simulink model "control_system"  (R2020b)
settings: Solver=FixedStepAuto  StartTime=0.0  StopTime=t_sim  FixedStep=Ts  RelTol=1e-2
values from neighbouring files (symbols this model uses):
  Hp = 10    [main_script.m]
  InitPosX = -2.4980e+03    (= -2498)    [main_script.m]
  InitPosY = -650.5503    [main_script.m]
  InitVelX = V0*cosd(InitYaw)    [main_script.m]
  InitVelY = V0*sind(InitYaw)    [main_script.m]
  InitYaw = 21    [main_script.m]
  lr = 1.592    [main_script.m]
  m = 1625    [main_script.m]
  Ts = 0.1    [main_script.m]
  V0 = 25    [main_script.m]
libraries: neural x856, simulink x1, autolibshared x1, drivingscenarioandsensors x1
(part 40 of 40)

== system control_system/HK con span dati 50 50 /Layer 3/Delays 1 ==
  "p{3}" : Inport  PortDimensions=50  SampleTime=0.1
      mask Display: e = 0.06;c1 = [120 230 180]/255;c2 = ([120 230 180]+0)/(256+128);c3 = ([120 230 180]+128)/(256+128);patch([0 1 1 0],[0 0 1 1],c1);patch([0 1 1 1-e 1-e 0+e],[0 0 1 1-e 0+e 0+e],c2);patch([0 0 1 1-e 0+e 0+e],[0 1 1 1-e 1-e 0+e],c3);plot([0 1 1 0 0],[0 0 1 1 0]);
  mux : Mux  Inputs=1
      mask Display: e = 0.06;c1 = [120 150 230]/255;c2 = ([120 150 230]+0)/383;c3 = ([120 150 230]+128)/383;patch([0 1 1 0],[0 0 1 1],c1);patch([0 1 1 1-e 1-e 0+e],[0 0 1 1-e 0+e 0+e],c2);patch([0 0 1 1-e 0+e 0+e],[0 1 1 1-e 1-e 0+e],c3);plot([0 1 1 0 0],[0 0 1 1 0]);disp('Mux')
  "pd{3,2}" : Outport
      mask Display: e = 0.06;c1 = [120 230 180]/255;c2 = ([120 230 180]+0)/(256+128);c3 = ([120 230 180]+128)/(256+128);patch([0 1 1 0],[0 0 1 1],c1);patch([0 1 1 1-e 1-e 0+e],[0 0 1 1-e 0+e 0+e],c2);patch([0 0 1 1-e 0+e 0+e],[0 1 1 1-e 1-e 0+e],c3);plot([0 1 1 0 0],[0 0 1 1 0]);
  wires:
  "p{3}"/1 -> mux/1
  mux/1 -> "pd{3,2}"/1

== system control_system/HK con span dati 50 50 /Layer 3/LW{3,2} ==
  "ad{3,2}" : Inport  PortDimensions=50  SampleTime=0.1
      mask Display: e = 0.06;c1 = [120 230 180]/255;c2 = ([120 230 180]+0)/(256+128);c3 = ([120 230 180]+128)/(256+128);patch([0 1 1 0],[0 0 1 1],c1);patch([0 1 1 1-e 1-e 0+e],[0 0 1 1-e 0+e 0+e],c2);patch([0 0 1 1-e 0+e 0+e],[0 1 1 1-e 1-e 0+e],c3);plot([0 1 1 0 0],[0 0 1 1 0]);
  "IW{3,2}(1,:)'" : Constant  Value=[-3.53332826646673137105381101719103753566741943359375;0.291507037926716783271530175625230185687541961669921875;-0.353172688693744574184307793984771706163883209228515625;-1.6395166117947235218110790810897015035152435302734375;0.50878764421372524306974582941620610654354095458984375;-0.5480368977260765550596488537848927080631256103515625;0.552184856715687288897242979146540164947509765625;0.76081482289424140486033820707234553992748260498046875;0.370219705857955216909971341010532341897487640380859375;1.6866898293792775831434482824988663196563720703125;0.46041883039566100510597834727377630770206451416015625;0.293600086588905295759133196042967028915882110595703125;0.438868226588818688416182567380019463598728179931640625;0.71701414029024979068793754777288995683193206787109375;0.60074691622149301029054413447738625109195709228515625;0.360264149329229510509975398235837928950786590576171875;0.34807246412229553289563455109600909054279327392578125;0.1417371042032999628457190510744112543761730194091796875;0.2504625689834882873441301853745244443416595458984375;-0.37020479133339201371910576199297793209552764892578125;-0.346173859388357929578461380515363998711109161376953125;0.3405441513736524594690990852541290223598480224609375;-0.34088615645206521431731516713625751435756683349609375;-0.179812084794879201155026748892851173877716064453125;0.1998575322053002534250509825142216868698596954345703125;-0.2200538783486616078999276169270160607993602752685546875;1.640532886970199388798619111184962093830108642578125;0.186500178645137515420771023855195380747318267822265625;0.5071129724580607511796870312537066638469696044921875;0.08063920908443254764730312444953597150743007659912109375;-0.306927876349457673388343437181902118027210235595703125;0.6080823360766220986306507256813347339630126953125;0.2892945314898811570714087793021462857723236083984375;-0.1795861371313421661621845260015106759965419769287109375;0.3366900876707565881673644980764947831630706787109375;-0.60768828590126344746380482320091687142848968505859375;-0.1801845560207073759784179856069386005401611328125;0.20445768532080810242490542805171571671962738037109375;-0.311847366447380258680510678459540940821170806884765625;0.2158239417458625852841436199014424346387386322021484375;2.1907776163678907010989860282279551029205322265625;0.2482784684639368910641366028357879258692264556884765625;0.64184501918167813361293383422889746725559234619140625;0.37579121007342031202114185362006537616252899169921875;-0.21851869728468098497131677504512481391429901123046875;-0.2276966088677858379707430458438466303050518035888671875;-3.356449993447315538475095308967866003513336181640625;3.484749592622747638159808047930710017681121826171875;-1.8624140445228880569317198023782111704349517822265625;2.150511605753588018075106447213329374790191650390625]
      mask Display: e = 0.06;c1 = [120 150 230]/255;c2 = ([120 150 230]+0)/383;c3 = ([120 150 230]+128)/383;patch([0 1 1 0],[0 0 1 1],c1);patch([0 1 1 1-e 1-e 0+e],[0 0 1 1-e 0+e 0+e],c2);patch([0 0 1 1-e 0+e 0+e],[0 1 1 1-e 1-e 0+e],c3);plot([0 1 1 0 0],[0 0 1 1 0]);disp('weights');
  Mux : Mux  Inputs=1
      mask Display: e = 0.06;c1 = [120 150 230]/255;c2 = ([120 150 230]+0)/383;c3 = ([120 150 230]+128)/383;patch([0 1 1 0],[0 0 1 1],c1);patch([0 1 1 1-e 1-e 0+e],[0 0 1 1-e 0+e 0+e],c2);patch([0 0 1 1-e 0+e 0+e],[0 1 1 1-e 1-e 0+e],c3);plot([0 1 1 0 0],[0 0 1 1 0]);disp('Mux');
  dotprod1 : neural/Weight Functions/dotprod
  "lz{3,2}" : Outport
      mask Display: e = 0.06;c1 = [120 230 180]/255;c2 = ([120 230 180]+0)/(256+128);c3 = ([120 230 180]+128)/(256+128);patch([0 1 1 0],[0 0 1 1],c1);patch([0 1 1 1-e 1-e 0+e],[0 0 1 1-e 0+e 0+e],c2);patch([0 0 1 1-e 0+e 0+e],[0 1 1 1-e 1-e 0+e],c3);plot([0 1 1 0 0],[0 0 1 1 0]);
  wires:
  "IW{3,2}(1,:)'"/1 -> dotprod1/1
  "ad{3,2}"/1 -> dotprod1/2
  dotprod1/1 -> Mux/1
  Mux/1 -> "lz{3,2}"/1

== matlab function control_system/scenario and environment/Pack Ego Actor ==
  data: pos input; a output Bus: BusActors1Actors size=1; vel input; yaw input; yawRate input
function a = packEgo(pos,vel,yaw,yawRate)
% Pack ego information into a single ego actor bus
%
% Imoprtant note:
% Output is a bus of type BusActorsActors. This is the same bus used by the
% Scenario Reader to output an individual actor. If you change the
% output bus name of Scenario Reader change the output bus name here
% as well by clicking on 'Edit Data' in the menu above.

a = struct(...
    'ActorID',1,...
    'Position', [pos(1) pos(2) 0], ...
    'Velocity', [vel(1) vel(2) 0], ...
    'Roll', 0, ...
    'Pitch', 0, ...
    'Yaw', yaw, ...
    'AngularVelocity', [0 0 yawRate]);

== matlab function control_system/MATLAB Function2 ==
  data: lanes input; latOff_1 output; latOff_2 output; latOff_3 output; latOff_4 output
function [latOff_1,latOff_2,latOff_3,latOff_4] = fcn(lanes)

latOff_1 = lanes.LaneBoundaries(1).LateralOffset;
latOff_2 = lanes.LaneBoundaries(2).LateralOffset;
latOff_3 = lanes.LaneBoundaries(3).LateralOffset;
latOff_4 = lanes.LaneBoundaries(4).LateralOffset;

== matlab function control_system/MATLAB Function6 ==
  data: steer_ang_deg input; acc_pedal_perc output; acc_m_s2 input; brake_pedal_perc output; steer_wheel_deg output
function [acc_pedal_perc,brake_pedal_perc,steer_wheel_deg] = actuators(steer_ang_deg,acc_m_s2)

steer_ratio = 15;
max_acc = 2;
max_dec = 3;

steer_wheel_deg = steer_ang_deg*steer_ratio;

acc_pedal_perc = 0;
brake_pedal_perc = 0;

if acc_m_s2 >= 0
    acc_pedal_perc = abs(acc_m_s2/max_acc)*100;
else
    brake_pedal_perc = abs(acc_m_s2/max_dec)*100;
end

== matlab function control_system/MATLAB Function4 ==
  data: lane_info input; k_hook input; x0 input; LAT_state input; LON_state input; LaneDet input; ObjDet input; X_opt input; InLK output size=22; InHK output size=26; InOT output size=22; InRE output size=22; OutLK output size=2; OutHK output size=2; OutOT output size=2; OutRE output size=2; vdes input
function [InLK,InHK,InOT,InRE,OutLK,OutHK,OutOT,OutRE] = IO_NN( lane_info, k_hook, x0, ...
    LAT_state, LON_state, LaneDet,ObjDet,X_opt,vdes)

%% INITIALIZATION
% if the Net is disabled both Out and In are set to 0

N_line = 4-lane_info(1)+1;
Curv = LaneDet.LaneBoundaries(N_line).Curvature(end);

num_coord = 4:6;
nR = 22;%8+num_coord*4+1;
 
OutLK = zeros(2,1);
OutHK = zeros(2,1);
OutOT = zeros(2,1);
OutRE = zeros(2,1);

InLK = zeros(nR,1);
InHK = zeros(nR+4,1);
InOT = zeros(nR,1);
InRE = zeros(nR,1);

%% TAKING MEASURES
if lane_info(3) == 1
    if(lane_info(1) == lane_info(2))
        LL = 4-lane_info(2);
        RL = 4-lane_info(1)+2;
    else 
        LL = 4-lane_info(2);
        RL = 4-lane_info(1)+1;
    end
    
elseif lane_info(3) == -1
        if(lane_info(1) == lane_info(2))
            LL = 4-lane_info(1)-1;
            RL = 4-lane_info(2)+1;
        else
            LL = 4-lane_info(1);
            RL = 4-lane_info(2)+1;
        end
else
    LL = 4-lane_info(2);
    RL = 4-lane_info(1)+1;
end


wall_measures = [LaneDet.LaneBoundaries(LL).Coordinates(num_coord,1)
                 LaneDet.LaneBoundaries(LL).Coordinates(num_coord,2)
                 LaneDet.LaneBoundaries(RL).Coordinates(num_coord,1)
                 LaneDet.LaneBoundaries(RL).Coordinates(num_coord,2)];
             
if k_hook ~= 0        
    Obs_measures = [ObjDet.Actors(k_hook).Position(1);
                    ObjDet.Actors(k_hook).Position(2);
                    ObjDet.Actors(k_hook).Velocity(1);
                    ObjDet.Actors(k_hook).Velocity(2)];
else
    Obs_measures = zeros(4,1);
end


if LON_state == 2
    if LAT_state == 2
        % LANE KEEPING NN
        InLK = [x0;
                vdes;
                wall_measures;
                Curv];
        OutLK = [X_opt(1,1);
                 X_opt(1,2)];
            
%     elseif LAT_state == 3
%         % OVERTAKE NN
%         InOT = [x0;
%                 t0;
%                 wall_measures;
%                   Curv];
%         OutOT = [X_opt(1,1);
%                 X_opt(1,2)];
%             
%     elseif LAT_state == 4
%         % RE-ENTRY NN
%         InRE = [x0;
%                 t0;
%                 wall_measures;
%                   Curv];
%         OutRE = [X_opt(1,1);
%                 X_opt(1,2)];
    end
    
elseif LON_state == 3
    % HOOKING NN
    InHK = [x0;
            vdes;
            wall_measures;
            Obs_measures;
                  Curv];
    OutHK = [X_opt(1,1);
             X_opt(1,2)];
end

== matlab function control_system/MATLAB Function5 ==
  data: LatState input; LonState input; en1 output; en2 output; en3 output; en4 output
function [en1,en2,en3,en4] = enable_funct(LatState,LonState)
% Finite-state machine for the lateral dynamics

% states:       "IDLE"  = [0]do nothing
%                "RST"  = [1]reset variables
%       "lane_keeping"  = [2]Lane keeping 
%         "overtaking"  = [3]move in the next left lane
%           "re_entry"  = [4]move in the next right lane

% Finite-state machine for the longitudinal dynamics

% states:       "IDLE"  = [0]do nothing
%                "RST"  = [1]reset variables
%           "vel_cntr"  = [2]velocity control
%            "hooking"  = [3]spacing control

en1 = 0;
en2 = 0;
en3 = 0;
en4 = 0;

if(LatState == 2 && LonState == 2)
    % classical Lane keeping
    en1 = 1;

elseif(LatState == 2 && LonState == 3)
    % Hooking + LK
    en2 = 1;
    
elseif(LatState == 3 && LonState == 2)
    % Overtake
    en3 = 1;
    
elseif(LatState == 4 && LonState == 2)
    % Re-entry
    en4 = 1;
end

== matlab function control_system/MATLAB Function7 ==
  data: en_NN1 output; LaneDet input; lane_info input; en_NN2 output
function [en_NN1, en_NN2] = Decisore(LaneDet,lane_info)

% en_NN1  = abilita NN per rettilineo e curva a sx
% en_NN2  = abilita NN per curva a dx

N_line = 4-lane_info(1)+1;
Curv = LaneDet.LaneBoundaries(N_line).Curvature(end);

if Curv >= 0 
    
   en_NN1 = 1;
   en_NN2 = 0;
   
else

   en_NN2 = 1;
   en_NN1 = 0;
   
end

== matlab function control_system/MATLAB Function8 ==
  data: InHK input; y output
function y = fcn(InHK)

y1 = InHK(1:21);
y2 = InHK(end);

y  = [y1;y2];

== matlab function control_system/MATLAB Function9 ==
  data: InHK input; in output
function in = fcn(InHK)

    x0   = InHK(4);
    pobs =  sqrt(InHK(22)^2+InHK(23)^2);
    vobs =  sqrt(InHK(24)^2+InHK(25)^2);
    
    in = [x0;vobs;pobs];

== matlab function control_system/MATLAB Function10 ==
  data: InHK input; y output
function y = fcn(InHK)

x0 = InHK(1:8);
vdes = InHK(9);
obs = InHK(22:25);

y = [x0;vdes;obs];

== matlab function control_system/MATLAB Function1 ==
  data: X_opt input; Acceleration output; dsteering_angle output
function [Acceleration,dsteering_angle] = fcn(X_opt)
Acceleration = X_opt(1,1);
dsteering_angle = X_opt(1,2)*0.1*180/pi;

== matlab function control_system/Controller/MPC_cntr ==
  settings: updateMethod=DISCRETE
  data: egoState input; LaneDet input; ObjDet input; v_ref_kmh input; acc_prev input; prev_curr_lane input; prev_lane_change input; steerAng_rad output size=1; x0 output; acc_m_s2 output size=1; current_lane output size=1; next_lane output; lane_change output; act_state_LAT output; prev_state_LAT input; act_state_LON output size=1; prev_state_LON input; prev_X_opt input; X_opt output; prev_flag_lane input; flag_lane output; k_hook output; t0_new output; t0 input; EFLAG output; v_des output
function [steerAng_rad,x0,acc_m_s2,current_lane,next_lane,lane_change,...
    act_state_LAT,act_state_LON,X_opt,flag_lane,k_hook,t0_new,EFLAG,v_des] = MPC(egoState,...
    LaneDet,ObjDet,v_ref_kmh,acc_prev,prev_curr_lane,prev_lane_change,...
    prev_state_LAT,prev_state_LON,prev_X_opt,prev_flag_lane,t0)

% ********** DEBUG ***********
%coder.extrinsic('optimizer');
% ****************************

%% INITIALIZATION DATA
v_ref_ms = v_ref_kmh/3.6;

Hp = 10;
Ts = 0.1;

% Headway time
head_t = 1.5;

% 0-speed safety distance
S0 = 2; % m

k_hook = 0;

% Vehicle specifications
VehData.Cf = 12000*2; %N/rad    %Cornering stiffness of the tyre
VehData.Cr = 11000*2; %N/rad

VehData.m = 1625;               % Mass of the Ego
VehData.Iz = 2865.61;           % Inertia in the Yaw axis

VehData.lr = 1.592;             % Axle lengths
VehData.lf = 1.108;

VehData.ego_L = 4.5; %m         % Ego length
VehData.L_wb = 1.7;             % Wheel base

% Comfort constraints
% Acceleration m/s^2
Con_acc.acc_max = 2;
Con_acc.acc_min = -3;
Con_acc.acc_lat_max = 1.5;
Con_acc.acc_lat_min = -1.5;

% Jerk m/s^3
Con_jrk.jerk_max = 2.5; %3.7
Con_jrk.jerk_min = -2.5; %-0.9
Con_jrk.jerk_lat_max = 1.8;
Con_jrk.jerk_lat_min = -1.8;

% Weight matrices
opt_mat.Ql      = 1*ones(1,Hp);
opt_mat.Qo      = 1*ones(1,Hp);
opt_mat.Qdv     = 0.1*eye(Hp); %0.2
opt_mat.Qddelta = 200*eye(Hp); %100
opt_mat.Qv      = 0.1*eye(Hp); %0.1
opt_mat.Qd      = 1*eye(Hp);

% Constraint on velocity
N_line = 4-prev_curr_lane+1;
Curv = LaneDet.LaneBoundaries(N_line).Curvature(end);

%Coordinate dei punti retta
v_max = 130/3.6;
v_min = 80/3.6;
P_A=[0,v_max];
P_B=[2e-3,v_min];

%Velocità di reference curvatura
v_ref_c_ms =(P_A(2)-P_B(2))/(P_A(1)-P_B(1))*(abs(Curv)-P_A(1))+P_A(2);

v_ref_c_ms = min([v_ref_ms, v_ref_c_ms, sqrt(Con_acc.acc_lat_max./abs(Curv))]);

% Velocity vector without taking into account the Yaw rotation wrt world
% frame
egoVel_NR = egoState.Velocity;

% Rotation (rototranslation) matrix to take into account the Yaw rotation
R = [cosd(egoState.Yaw) sind(egoState.Yaw) 0;
    -sind(egoState.Yaw) cosd(egoState.Yaw) 0;
    0 0 1];

% Velocity vector correctly rotated
egoVel = egoVel_NR*R'; 

% ----- Ego vehicle oriented wrt world frame (0,0) -----

% x-speed component 
v0x = egoVel(1);

% y-speed component
v0y = egoVel(2); 

% total speed
v0 = sqrt(v0x^2+v0y^2); 

% yaw rate [rad/s]
w0 = egoState.AngularVelocity(3)*pi/180; 

% Actual steering angle [rad]
delta0 = atan2(w0*VehData.ego_L/v0x,1);

% for each iteration the state become the initial state
x0 = [0;0;0;v0;delta0;v0y;v0x;w0];

%NB: This approach try to solve the problem of the curvature of the road,
%by rotating step-by-step the vehicle reference frame in order to 
%keep the 0 yaw orientation

X_opt = prev_X_opt;

u0=[X_opt(2:end,:); X_opt(end,:)];

%% FSM longitudinal state / lateral state

[next_lane,current_lane,lane_change,v_ref_c_ms,k_closest,...
    next_state_LAT,next_state_LON,flag_lane] = perception(prev_state_LAT,...
    v_ref_c_ms,egoState,R,ObjDet,LaneDet,prev_curr_lane,...
    prev_lane_change,x0,prev_flag_lane,head_t,S0);

% Finite-state machine for the lateral dynamics

% states:       "IDLE"  = [0]do nothing
%                "RST"  = [1]reset variables
%       "lane_keeping"  = [2]Lane keeping 
%         "overtaking"  = [3]move in the next left lane
%           "re_entry"  = [4]move in the next right lane

% Finite-state machine for the longitudinal dynamics

% states:       "IDLE"  = [0]do nothing
%                "RST"  = [1]reset variables
%           "vel_cntr"  = [2]velocity control
%            "hooking"  = [3]spacing control


% UPDATE STATE LATERAL DYNAMICS ------------------------------------------

switch(prev_state_LAT)
    
    case 0 % IDLE
        next_state_LAT = 1;
    
    case 1 % RST 
        next_state_LAT = 2;
        
    case 2 % LANE KEEPING
        
    case 3 % OVERTAKE
         
    case 4 % RE-ENTRY
        
    otherwise
        next_state_LAT = 1;
end

act_state_LAT = next_state_LAT;

% UPDATE STATE LONGITUDINAL DYNAMICS -------------------------------------

switch(prev_state_LON)
    
    case 0 % IDLE
        next_state_LON = 1;
        
    case 1 % RST
        next_state_LON = 2;
        
    case 2 % VELOCITY CONTROL
         
    case 3 % SPACING CONTROL
             
    otherwise
        next_state_LON = 1;
end

act_state_LON = next_state_LON;
        
% UPDATE OUTPUT LATERAL DYNAMICS -----------------------------------------

switch(act_state_LAT)
    
    case 1 % RST
        % reset all the variables
        
    case 2 % LANE KEEPING
        
    case 3 % OVERTAKE
        % Disable the obstacle cost
        opt_mat.Qd = 0*eye(Hp);
        opt_mat.Qdv = 1*eye(Hp);
        
        
    case 4 % RE-ENTRY
        % Disable the obstacle cost
        opt_mat.Qd = 0*eye(Hp);
        opt_mat.Qdv = 1*eye(Hp);
        
    otherwise
        % do-nothing
end

% UPDATE OUTPUT LONGITUDINAL DYNAMICS ------------------------------------

switch(act_state_LON)
    
    case 1 % RST
        % reset all the variables
        
    case 2 % VELOCITY CONTROL
       
        % During the speed control the controller doesn't keep into account
        % the eventual vehicle in front
         opt_mat.Qd = 0*eye(Hp);
        
    case 3 % DISTANCE CONTROL
        
        % During the distance control the system use the maximum
        % acceleration possible (anyway constrained)
        opt_mat.Qv = 0*eye(Hp);
        opt_mat.Qdv = 0.02*eye(Hp);
             
    otherwise
        % do-nothing
end

%% OUTPUT COMPUTATION

% Optimization process
%tic
[t0_new,X_opt,EFLAG,v_des] = optimizer(opt_mat,Con_acc,Con_jrk,...
acc_prev,VehData,Ts,egoState,ObjDet,LaneDet,current_lane,next_lane,...
lane_change,k_closest,head_t,S0,v_ref_c_ms,Hp,x0,u0,R,t0,next_state_LON);
% toc
if ~isempty(k_closest)
    k_hook = k_closest(1);
end

% Rounding results
%X_opt(:,1)=round(X_opt(:,1)*100)/100;
%X_opt(:,2)=round(X_opt(:,2)*1000)/1000;

% Steering angle output
steerAng_rad = X_opt(1,2)*Ts;

% Acceleration output
% If the problem is infeasible for the hooking, brake manually
if(EFLAG < 0 && next_state_LON == 3) 
    X_opt(:,1) = acc_prev+Con_jrk.jerk_min*Ts;
end
    acc_m_s2 = X_opt(1,1);

== matlab function control_system/MATLAB Function3 ==
  data: LaneDet input; Curv_end output
function Curv_end = fcn(LaneDet)

Curv_end = LaneDet.LaneBoundaries(1).Curvature(end);

== matlab function control_system/MATLAB Function ==
  data: lanes input; err_lane_sx output; err_lane_dx output
function [err_lane_sx,err_lane_dx] = fcn(lanes)

err_lane_sx = lanes.LaneBoundaries(3).LateralOffset - 1.75;
err_lane_dx = lanes.LaneBoundaries(4).LateralOffset + 1.75;
